simulink model "PD_controller"  (R2025b)
settings: Solver=VariableStepAuto  StartTime=0.0  StopTime=10  RelTol=1e-3
settings Model: Creator=sengu  LastModifiedBy=sengu

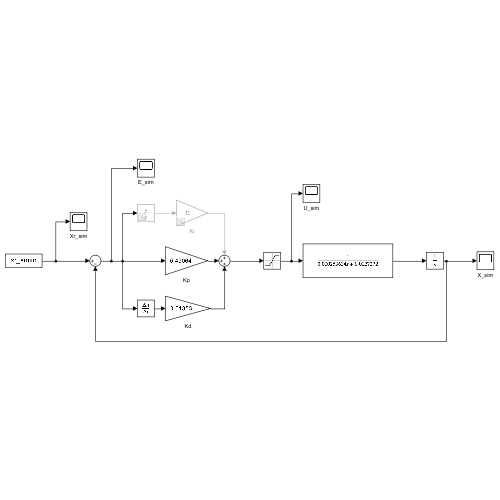
[thumbnail: Simulink's stored preview of the top-level diagram]
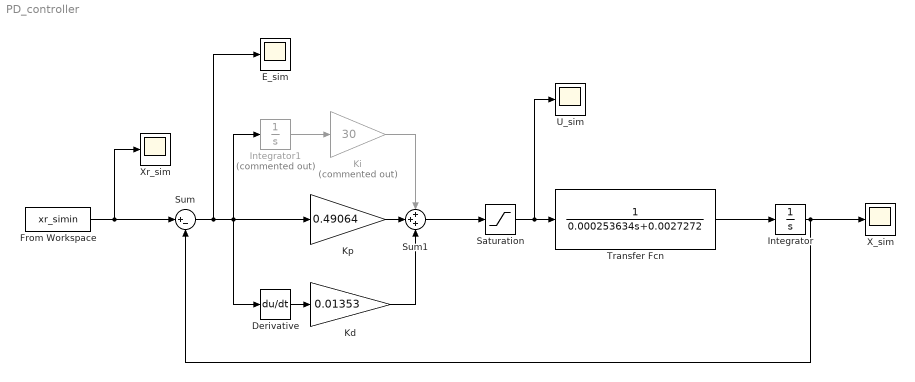
== system PD_controller ==
  Derivative : Derivative
  E_sim : Scope
      settings: ActiveDisplayYMinimum=-0.010277611876142536  ActiveDisplayYMaximum=0.05129796457847359  DataLoggingVariableName=e_sim  DataLoggingSaveFormat=Array
  From Workspace : FromWorkspace  VariableName=xr_simin
  Integrator : Integrator
  Integrator1 : Integrator  Commented=on
  Kd : Gain  Gain=0.01353
  Ki : Gain  Commented=on  Gain=30
  Kp : Gain  Gain=0.49064
  Saturation : Saturate  UpperLimit=10  LowerLimit=-10
  Sum : Sum  Inputs=|+-
  Sum1 : Sum  Inputs=+++
  Transfer Fcn : TransferFcn  Denominator=[0.000253634 0.0027272]
  U_sim : Scope
      settings: ActiveDisplayYMinimum=-0.48060153644248227  ActiveDisplayYMaximum=0.48106144397274281  DataLoggingVariableName=u_sim  DataLoggingSaveFormat=Array
  X_sim : Scope
      settings: ActiveDisplayYMinimum=-2.6033865969925345  ActiveDisplayYMaximum=2.5786015903640132  DataLoggingVariableName=x_sim  DataLoggingSaveFormat=Array
  Xr_sim : Scope
      settings: ActiveDisplayYMinimum=-6.2499999999999982  ActiveDisplayYMaximum=56.25  DataLoggingVariableName=xr_sim  DataLoggingSaveFormat=Array
  wires:
  From Workspace/1 -> Xr_sim/1, Sum/1
  Sum/1 -> E_sim/1, Integrator1/1, Derivative/1, Kp/1
  Kp/1 -> Sum1/2
  Sum1/1 -> Saturation/1
  Derivative/1 -> Kd/1
  Saturation/1 -> U_sim/1, Transfer Fcn/1
  Transfer Fcn/1 -> Integrator/1
  Integrator/1 -> Sum/2, X_sim/1
  Kd/1 -> Sum1/3
  Ki/1 -> Sum1/1
  Integrator1/1 -> Ki/1
